simulink model "msbr_pke_circ"  (R2015b)
settings: Solver=ode45  StartTime=0.0  StopTime=simtime  RelTol=1e-3
values from neighbouring files (symbols this model uses):
  beta = [2.290E-04, 8.320E-04, 7.100E-04, 8.520E-04, 1.710E-04, 1.020E-04]    [Parameters_Core_PHE.m]    (also in Parameters_Core_PHE_FEHE.m; Parameters_MSBR.m; parameters_msbr_pke_circ.m = [0.000215, 0.00142, 0.00127, 0.00257, 0.00075, 0.00027]; parameters_msbr_pke_stat.m)
  beta_t = sum(beta)    [Parameters_Core_PHE.m]    (also in Parameters_Core_PHE_FEHE.m; Parameters_MSBR.m; parameters_msbr_pke_circ.m; parameters_msbr_pke_stat.m = 0.002896)
  C0 = lam.\beta/Lam    [parameters_msbr_pke_stat.m]
  Lam = 3.300E-04    (= 0.00033)    [Parameters_Core_PHE.m]    (also in Parameters_Core_PHE_FEHE.m; Parameters_MSBR.m; parameters_msbr_pke_circ.m; parameters_msbr_pke_stat.m)
  lam = [1.260E-02, 3.370E-02, 1.390E-01, 3.250E-01, 1.130E+00, 2.500E+00]    [Parameters_Core_PHE.m]    (also in Parameters_Core_PHE_FEHE.m; Parameters_MSBR.m; param.m = [0.0126, 0.0337, 0.139, 0.325, 1.13, 2.50]'; parameters_msbr_pke_circ.m = [0.0126, 0.0337, 0.139, 0.325, 1.13, 2.50])
  n_frac0 = 1    [Parameters_Core_PHE.m]    (also in Parameters_Core_PHE_FEHE.m; Parameters_MSBR.m; parameters_msbr_pke_circ.m; parameters_msbr_pke_stat.m)
  rho_0 = beta_t - bigterm(beta,lam,Lam,tau_l,tau_c)    [Parameters_Core_PHE.m]    (also in Parameters_Core_PHE_FEHE.m; Parameters_MSBR.m; bigterm.m = rho_0 + bet(i)/(1.0 + (1.0-exp(-lam(i)*t_L))/(lam(i)*t_C)); parameters_msbr_pke_circ.m)
  tau_c = 3.28    [Parameters_Core_PHE.m]    (also in Parameters_Core_PHE_FEHE.m; Parameters_MSBR.m; parameters_msbr_pke_circ.m)
  tau_l = 5.85    [Parameters_Core_PHE.m]    (also in Parameters_Core_PHE_FEHE.m; Parameters_MSBR.m; parameters_msbr_pke_circ.m)
libraries: simulink x1
settings Model: Creator=mlish  LastModifiedBy=mlish
settings DataIOCC: LimitDataPoints=off

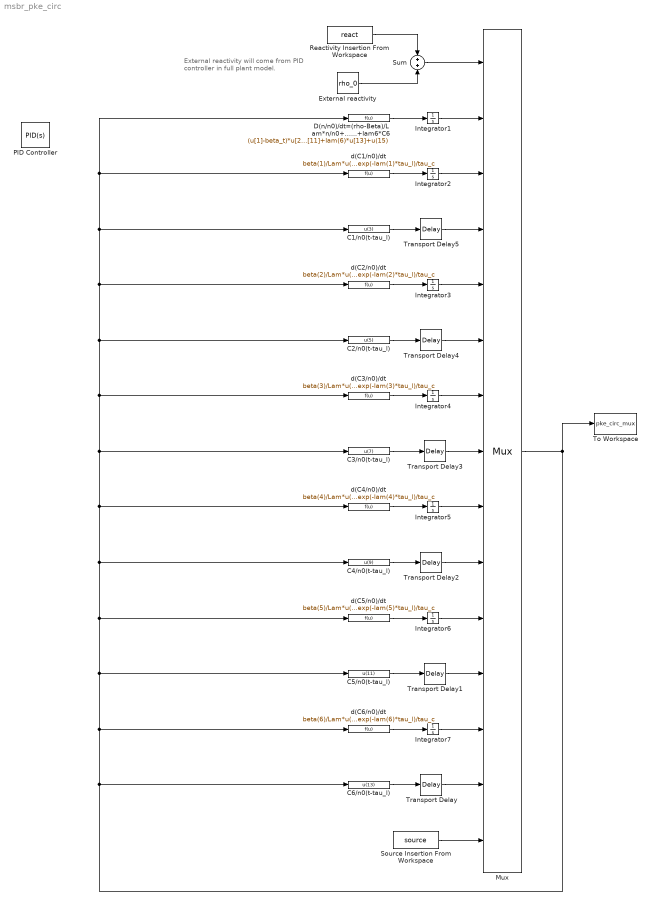
== system msbr_pke_circ ==
  note: External reactivity will come from
      | PID controller in full plant model.
  C1/n0(t-tau_l) : Fcn  Expr=u(3)
  C2/n0(t-tau_l) : Fcn  Expr=u(5)
  C3/n0(t-tau_l) : Fcn  Expr=u(7)
  C4/n0(t-tau_l) : Fcn  Expr=u(9)
  C5/n0(t-tau_l) : Fcn  Expr=u(11)
  C6/n0(t-tau_l) : Fcn  Expr=u(13)
  D(n/n0)/dt=(rho-Beta)/Lam*n/n0+lam1*C1+...+lam6*C6 : Fcn  Expr=(u[1]-beta_t)*u[2]/Lam+lam(1)*u[3]+lam(2)*u[5]+lam(3)*u[7]+lam(4)*u[9]+lam(5)*u[11]+lam(6)*u[13]+u(15)
  External reactivity : Constant  Value=rho_0
  Integrator1 : Integrator  InitialCondition=n_frac0
  Integrator2 : Integrator  InitialCondition=C0(1)
  Integrator3 : Integrator  InitialCondition=C0(2)
  Integrator4 : Integrator  InitialCondition=C0(3)
  Integrator5 : Integrator  InitialCondition=C0(4)
  Integrator6 : Integrator  InitialCondition=C0(5)
  Integrator7 : Integrator  InitialCondition=C0(6)
  Mux : Mux  Inputs=15
      settings: DisplayOption=signals
  PID Controller : simulink/Continuous/PID Controller  Controller=PID  TimeDomain=Continuous-time  SampleTime=-1  IntegratorMethod=Forward Euler  FilterMethod=Forward Euler  Form=Parallel  UseFilter=on  ControllerParametersSource=internal  P=0.00135357236899509  I=0.0215256947163999  D=-7.28028646852379e-05  N=6.58840916944279  InitialConditionSource=internal  InitialConditionForIntegrator=0  InitialConditionForFilter=0  ExternalReset=none  LimitOutput=off  UpperSaturationLimit=inf  LowerSaturationLimit=-inf  LinearizeAsGain=on  AntiWindupMode=none  Kb=1  TrackingMode=off  Kt=1  PParamMin=[]  PParamMax=[]  IParamMin=[]  IParamMax=[]  DParamMin=[]  DParamMax=[]  NParamMin=[]  NParamMax=[]  KbParamMin=[]  KbParamMax=[]  KtParamMin=[]  KtParamMax=[]  POutMin=[]  POutMax=[]  IOutMin=[]  IOutMax=[]  DOutMin=[]  DOutMax=[]  NOutMin=[]  NOutMax=[]  KbOutMin=[]  KbOutMax=[]  KtOutMin=[]  KtOutMax=[]  IntegratorOutMin=[]  IntegratorOutMax=[]  FilterOutMin=[]  FilterOutMax=[]  SumOutMin=[]  SumOutMax=[]  SumI1OutMin=[]  SumI1OutMax=[]  SumI2OutMin=[]  SumI2OutMax=[]  SumI3OutMin=[]  SumI3OutMax=[]  SumDOutMin=[]  SumDOutMax=[]  SaturationOutMin=[]  SaturationOutMax=[]  IntegratorContinuousStateAttributes=''  IntegratorStateMustResolveToSignalObject=off  IntegratorRTWStateStorageClass=Auto  FilterContinuousStateAttributes=''  FilterStateMustResolveToSignalObject=off  FilterRTWStateStorageClass=Auto  DifferentiatorICPrevScaledInput=0  DifferentiatorOutMin=[]  DifferentiatorOutMax=[]
  Reactivity Insertion From Workspace : FromWorkspace  VariableName=react  Interpolate=off  OutputAfterFinalValue=Holding final value
  Source Insertion From Workspace : FromWorkspace  VariableName=source  Interpolate=off  OutputAfterFinalValue=Holding final value
  Sum : Sum  Inputs=+|+
  To Workspace : ToWorkspace  VariableName=pke_circ_mux  SampleTime=-1
  Transport Delay : TransportDelay  DelayTime=tau_l  InitialOutput=C0(6)  BufferSize=4096
  Transport Delay1 : TransportDelay  DelayTime=tau_l  InitialOutput=C0(5)  BufferSize=4096
  Transport Delay2 : TransportDelay  DelayTime=tau_l  InitialOutput=C0(4)  BufferSize=4096
  Transport Delay3 : TransportDelay  DelayTime=tau_l  InitialOutput=C0(3)  BufferSize=4096
  Transport Delay4 : TransportDelay  DelayTime=tau_l  InitialOutput=C0(2)  BufferSize=4096
  Transport Delay5 : TransportDelay  DelayTime=tau_l  InitialOutput=C0(1)  BufferSize=4096
  d(C1/n0)/dt : Fcn  Expr=beta(1)/Lam*u(2)-lam(1)*u(3)-u(3)/tau_c+u(4)*exp(-lam(1)*tau_l)/tau_c
  d(C2/n0)/dt : Fcn  Expr=beta(2)/Lam*u(2)-lam(2)*u(5)-u(5)/tau_c+u(6)*exp(-lam(2)*tau_l)/tau_c
  d(C3/n0)/dt : Fcn  Expr=beta(3)/Lam*u(2)-lam(3)*u(7)-u(7)/tau_c+u(8)*exp(-lam(3)*tau_l)/tau_c
  d(C4/n0)/dt : Fcn  Expr=beta(4)/Lam*u(2)-lam(4)*u(9)-u(9)/tau_c+u(10)*exp(-lam(4)*tau_l)/tau_c
  d(C5/n0)/dt : Fcn  Expr=beta(5)/Lam*u(2)-lam(5)*u(11)-u(11)/tau_c+u(12)*exp(-lam(5)*tau_l)/tau_c
  d(C6/n0)/dt : Fcn  Expr=beta(6)/Lam*u(2)-lam(6)*u(13)-u(13)/tau_c+u(14)*exp(-lam(6)*tau_l)/tau_c
  wires:
  Mux/1 -> To Workspace/1, C6/n0(t-tau_l)/1, d(C6/n0)/dt/1, C5/n0(t-tau_l)/1, d(C5/n0)/dt/1, C4/n0(t-tau_l)/1, d(C4/n0)/dt/1, C3/n0(t-tau_l)/1, d(C3/n0)/dt/1, C2/n0(t-tau_l)/1, d(C2/n0)/dt/1, C1/n0(t-tau_l)/1, d(C1/n0)/dt/1, D(n/n0)/dt=(rho-Beta)/Lam*n/n0+lam1*C1+...+lam6*C6/1
  D(n/n0)/dt=(rho-Beta)/Lam*n/n0+lam1*C1+...+lam6*C6/1 -> Integrator1/1
  d(C1/n0)/dt/1 -> Integrator2/1
  d(C2/n0)/dt/1 -> Integrator3/1
  d(C3/n0)/dt/1 -> Integrator4/1
  d(C4/n0)/dt/1 -> Integrator5/1
  d(C5/n0)/dt/1 -> Integrator6/1
  d(C6/n0)/dt/1 -> Integrator7/1
  Integrator1/1 -> Mux/2
  Integrator2/1 -> Mux/3
  Integrator3/1 -> Mux/5
  Integrator4/1 -> Mux/7
  Integrator5/1 -> Mux/9
  Integrator6/1 -> Mux/11
  Integrator7/1 -> Mux/13
  C6/n0(t-tau_l)/1 -> Transport Delay/1
  Transport Delay/1 -> Mux/14
  C5/n0(t-tau_l)/1 -> Transport Delay1/1
  Transport Delay1/1 -> Mux/12
  Transport Delay2/1 -> Mux/10
  C4/n0(t-tau_l)/1 -> Transport Delay2/1
  C3/n0(t-tau_l)/1 -> Transport Delay3/1
  Transport Delay3/1 -> Mux/8
  Transport Delay4/1 -> Mux/6
  C2/n0(t-tau_l)/1 -> Transport Delay4/1
  Transport Delay5/1 -> Mux/4
  C1/n0(t-tau_l)/1 -> Transport Delay5/1
  Source Insertion From Workspace/1 -> Mux/15
  Sum/1 -> Mux/1
  External reactivity/1 -> Sum/2
  Reactivity Insertion From Workspace/1 -> Sum/1
